simulink model "psb3levelVSC"  (Simulink 6.0)
settings: Solver=FixedStepDiscrete  SolverMode=SingleTasking  StartTime=0.0  StopTime=0.15  FixedStep=Ts_Power  RelTol=1e-3
PreLoadFcn:
  | assignin('base','Ts_Power',[5e-6]);assignin('base','Ts_Control',[100e-6])
undefined symbols (not defined in the file or in its folder): D1, Delta, gcbh, level, powericon, Ts_Control, Ts_Power
libraries: powerlib_extras x18, powerlib2 x17, simulink_extras x1
settings Model: Creator=sybille  LastModifiedBy=batserve  ExtModeTrigMode=oneshot  ExtModeArmWhenConnect=off  ExtModeAutoUpdateStatusClock=off  ProdHWDeviceType=Specified
settings DataIOCC: LimitDataPoints=off  SaveFormat=StructureWithTime  SaveOutput=off  SaveTime=off  SignalLoggingName=sigsOut
settings OptimizationCC: BlockReduction=off  BooleanDataType=off
settings DebuggingCC: SolverPrmCheckMsg=none
settings HardwareCC: ProdBitPerShort=32  ProdBitPerInt=16  ProdHWDeviceType=Specified  TargetUnknown=on

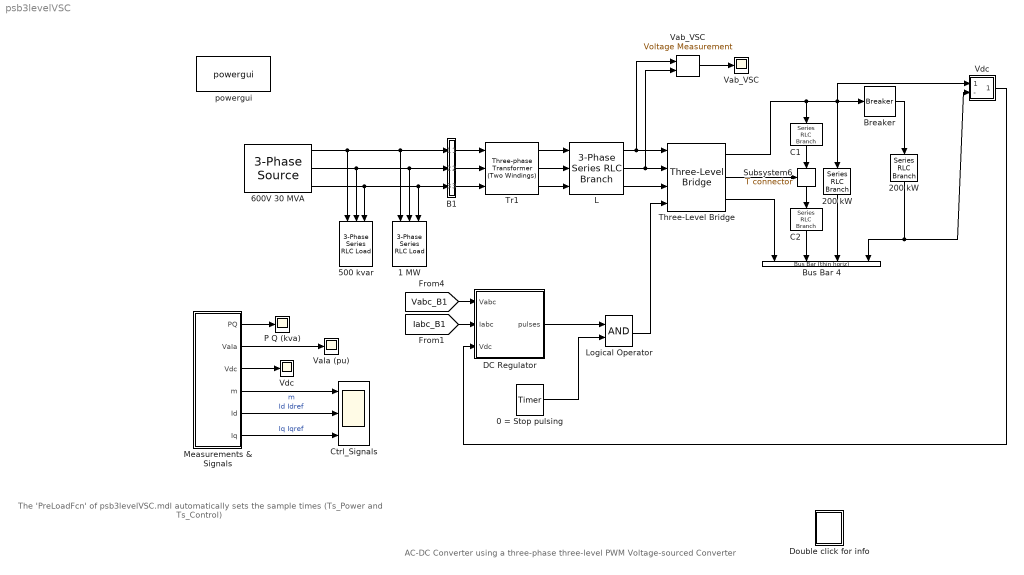
== system psb3levelVSC ==
  note: AC-DC Converter
      | using a three-phase three-level PWM Voltage-sourced Converter
  note: The 'PreLoadFcn' of psb3levelVSC.mdl automatically
      | sets the sample times (Ts_Power and Ts_Control)
  0 = Stop pulsing : powerlib_extras/Control  Blocks/Timer  t=[0 0.2]  e=[1 0]
  1 MW : powerlib2/Elements/3-Phase Series RLC Load  Orientation=down  Vpp=600  fn=60  P3=1e6  QL3=0  QC3=0
  200 kW : powerlib2/Elements/Series RLC Branch  Tag=PoWeRsYsTeMbLoCk  Orientation=down  a=500^2/200e3  b=0  c=inf  mesure=None  PSBOutputType=1
  "200 kW " : powerlib2/Elements/Series RLC Branch  Tag=PoWeRsYsTeMbLoCk  Orientation=down  a=500^2/200e3  b=0  c=inf  mesure=None  PSBOutputType=1
  500 kvar : powerlib2/Elements/3-Phase Series RLC Load  Orientation=down  Vpp=600  fn=60  P3=0.5e6/100  QL3=0  QC3=0.5e6
  600V 30 MVA : powerlib2/Electrical Sources/3-Phase Source  Tag=PoWeRsYsTeMbLoCk  V=600  Phi=0  F=60  InternalConnection=Yg  RLoff=on  R=0.724  L=19.2e-3  Psc=30e6  Vbase=600  XRratio=10  PSBOutputType=111
  B1 : Subsystem  Tag=PoWeRsYsTeMmEaSuReMeNt  AncestorBlock=powerlib2/Measurements/Three-Phase V-I Measurement  LoadFcn=powericon('psbloadfunction',gcbh,'3-Phase VI Measurement','');  InitFcn=powericon('checksum',bdroot)  mask(3-Phase VI Measurement){VChoice=phase-to-ground, ualv=on, labelV=Vabc_B1, Vpu=off, Vbase=500e3, IChoice=yes, ualc=on, labelC=Iabc_B1, Ppu=off, Pbase=100e6, OutputType=Magnitude, PhasorSimulation=off, PSBequivalent=0, PSBOutputType=11100}
      mask prompts: VChoice "Voltage measurement"; ualv "Use a label"; labelV "Signal label  (use a From block to collect signal)"; Vpu "Voltage  in pu"; Vbase "Base voltage (Vrms phase-phase) :"; IChoice "Current measurement"; ualc "Use a label"; labelC "Signal label  (use a From block to collect signal)"; Ppu "Currents in pu"; Pbase "Base power ( VA 3 phase)"; OutputType "Output signal :"; PhasorSimulation "Phasor simulation"; PSBequivalent "Equivalent circuit"
      mask help:
      | This block is used to measure three-phase voltages and currents in a circuit. When connected in series with a three-phase element, it return the three phase-to-ground voltages and line currents.
      |
      | The block can output the voltages and currents in per unit values or in volts and amperes. Check the appropriate boxes if you want to output the voltages and currents  in pu
      mask init:
      | powericon('psbcallbacks',gcb,'Three-phase measurements',4);
      | if  Vpu
      |     xKv=1/(Vbase/sqrt(3)*sqrt(2));
      | else
      |     xKv=1;
      | end
      | if  Ppu
      |     xKi=1/(Pbase/Vbase/sqrt(3)*sqrt(2));
      | else
      |     xKi=1;
      | end
      | switch OutputType
      | case 1
      |     OutputSelection  = [1:6];
      |     PhasorModeV = [1:3];
      |     NormalModeV = [7:9];
      |     PhasorModeI = [4:6];
      |     NormalModeI = [10:12];
      |     Kv = xKv;
      |     Ki = xKi;
      | case 2
      |     OutputSelection = [7,13,8,14,9,15,10,16,11,17,12,18];
      |     PhasorModeV = [1:6];
      |     NormalModeV = [13:15];
      |     PhasorModeI = [7:12];
      |     NormalModeI = [16:18];
      |     Kv = xKv;
      |     Ki = xKi;
      | case 3
      |     OutputSelection = [13,19,14,20,15,21,16,22,17,23,18,24];
      |     PhasorModeV = [1:6];
      |     NormalModeV = [13:15];
      |     PhasorModeI = [7:12];
      |     NormalModeI = [16:18];
      |     Kv = [xKv 1 xKv 1 xKv 1];
      |     Ki = [xKi 1 xKi 1 xKi 1];
      | case 4
      |     OutputSelection  = [19:24];
      |     PhasorModeV = [1:3];
      |     NormalModeV = [7:9];
      |     PhasorModeI = [4:6];
      |     NormalModeI = [10:12];
      |     Kv = xKv;
      |     Ki = xKi;
      | end
      | if PhasorSimulation
      |     SelectionModeV = PhasorModeV;
      |     SelectionModeI = PhasorModeI;
      | else
      |     SelectionModeV = NormalModeV;
      |     SelectionModeI = NormalModeI;
      |     Kv = xKv;
      |     Ki = xKi;
      | end
      settings: CopyFcn=powericon('psbloadfunction',gcbh,'3-Phase VI Measurement','VerifyPhasor');  CloseFcn=%3phaseVImeasurement
      mask Help: web(psbhelp)
      mask StyleString: popup(no|phase-to-ground|phase-to-phase),checkbox,edit,checkbox,edit,popup(no|yes),checkbox,edit,checkbox,edit,popup(Complex|Real-Imag|Magnitude-Angle|Magnitude),checkbox,edit,edit
      mask CallbackString: powericon('psbcallbacks',gcb,'Three-phase measurements',2);|powericon('psbcallbacks',gcb,'Three-phase measurements',2);||powericon('psbcallbacks',gcb,'Three-phase measurements',2);||powericon('psbcallbacks',gcb,'Three-phase measurements',2);|powericon('psbcallbacks',gcb,'Three-phase measurements',2);||powericon('psbcallbacks',gcb,'Three-phase measurements',4);|||||
  Breaker : powerlib2/Elements/Breaker  Tag=PoWeRsYsTeMbLoCk  a=0.001  c=0  rs=1e6  cs=inf  times=[0.15]  Ts=0  comext=off  mesure=None  PSBOutputType=1
  Bus Bar 4 : powerlib2/Connectors/Bus Bar (thin horiz)  Tag=PoWeRsYsTeMbLoCk  Orientation=down  input=4  output=0  PSBOutputType=111111111111111111111111111111111111111111111111111111111111111111111111111111111111
  C1 : powerlib2/Elements/Series RLC Branch  Tag=PoWeRsYsTeMbLoCk  Orientation=down  a=0  b=0  c=75000e-06  mesure=None  PSBOutputType=1
  C2 : powerlib2/Elements/Series RLC Branch  Tag=PoWeRsYsTeMbLoCk  Orientation=down  a=0  b=0  c=75000e-06  mesure=None  PSBOutputType=1
  Ctrl_Signals : Scope  NumInputPorts=3
      settings: YMin=0.6~-1~-1  YMax=1.2~1~1  SaveName=V_Load  DataFormat=Array  SampleInput=on  SampleTime=Ts_Control
  DC Regulator : Subsystem  mask(DC Voltage Regulator){Vdc_Ref=500}
      mask prompts: Vdc_Ref "DC voltage setpoint (V):"
  Double click for info : Subsystem
      mask Type: Information
      mask Display: disp('?')
  L : powerlib2/Elements/3-Phase Series RLC Branch   R=0.1e-3  L=20e-6  C=inf
  Logical Operator : Logic  AllPortsSameDT=off  OutDataTypeMode=Specify via dialog  LogicDataType=float('double')
  Measurements & Signals : Subsystem
  P Q (kva) : Scope
      settings: YMin=-25  YMax=425  SaveName=PQ  DataFormat=Array  SampleInput=on  SampleTime=Ts_Control
  Subsystem6 : powerlib2/Connectors/T connector  Tag=PoWeRsYsTeMbLoCk  Orientation=down  PSBOutputType=1
  Three-Level Bridge : powerlib2/Power Electronics/Three-Level Bridge  Tag=PoWeRsYsTeMbLoCk  arms=3  confi=ABC as input terminals  Rs=50  Cs=1e-6  device=IGBT / Diodes  Ron=0.2e-3  PAr_vf="[  2 1 ]"  mesure=All voltages and currents  PSBOutputType=111
  Tr1 : powerlib2/Elements/Three-phase Transformer (Two Windings)  Tag=PoWeRsYsTeMbLoCk  nominal=[ 500e3 , 60 ]  type1=Yg  params1=[ 600 , 0.04/30/2 , 0.04 ]  type2=Delta (D1)  params2=[ 240 , 0.04/30/2 , 0.0 ]  ynsat=off  rmag=500  lm=500  sat=[ 0,0 ; 0.0024,1.2 ; 1.0,1.52 ]  hyst=off  matfile='hysteresis'  sif=off  phi0=[ 0.8 , -0.8 , 0.7 ]  initialslopes=[+1 +1 +1]  mesure=None  PSBOutputType=1111
  VaIa (pu) : Scope
      settings: TimeRange=0.08  YMin=-2.5  YMax=1.5  SaveName=VaIa  SampleInput=on  SampleTime=Ts_Power*2
  Vab_VSC : Scope
      settings: TimeRange=0.05  YMin=-550  YMax=550  SaveName=Vab_VSC  SampleInput=on  SampleTime=Ts_Power
  "Vab_VSC " : powerlib2/Measurements/Voltage Measurement  Tag=PoWeRsYsTeMmEaSuReMeNt  PhasorSimulation=off  OutputType=Magnitude  PSBOutputType=0  PSBequivalent=0
  Vdc : Scope
      settings: YMin=200  YMax=600  SaveName=Vdc  DataFormat=Array  SampleInput=on  SampleTime=Ts_Control
  "Vdc " : Subsystem  Tag=PoWeRsYsTeMmEaSuReMeNt  AncestorBlock=powerlib2/Measurements/Voltage Measurement  LoadFcn=powericon('psblcfmeas',gcb)  InitFcn=powericon('checksum',bdroot)  mask(Voltage Measurement){PhasorSimulation=off, OutputType=Magnitude, PSBOutputType=0, PSBequivalent=0}
      mask prompts: PhasorSimulation "Phasor simulation"; OutputType "Output signal :"; PSBOutputType "Output type [1=PSB  0=simulink output]"; PSBequivalent "Equivalent circuit"
      mask help: Ideal voltage measurement.
      mask init:
      | switch OutputType
      | case 1
      |     OutputSelection = 1;
      |     NormalMode = 2;
      |     PhasorMode = 1;
      | case 2
      |     OutputSelection =[2,3];
      |     NormalMode = 3;
      |     PhasorMode = [1,2];
      | case 3
      |     OutputSelection =[4,5];
      |     NormalMode = 3;
      |     PhasorMode = [1,2];
      | case 4
      |     OutputSelection =[4];
      |     NormalMode = 2;
      |     PhasorMode = 1;
      | end
      | %
      | if PhasorSimulation
      |     SelectionMode = PhasorMode;
      | else
      |     SelectionMode = NormalMode;
      | end
      settings: CopyFcn=powericon('psblcfmeas',gcb,1)  ModelCloseFcn=powericon('loadsavedata',gcs,'close')
      mask Help: web(psbhelp);
      mask StyleString: checkbox,popup(Complex|Real-Imag|Magnitude-Angle|Magnitude),edit,edit
  powergui : powerlib2/powergui  Frange=logspace(0,3,50)  Ylog=off  Xlog=off  save=off  variable=ZData  structure=VaIa  ZoomFFT=on  StartTime=0.2  cycles=2  DisplayStyle=1  fundamental=60  FreqAxis=off  MaxFrequency=1000  frequencyindice=1  frequencyindicesteady=1  RmsSteady=2  display=off  Ts=Ts_Power  methode=off  frequency=60  echomessages=off
  wires:
  600V 30 MVA/1 -> B1/1(A), 1 MW/1, 500 kvar/1
  600V 30 MVA/2 -> B1/2(B), 1 MW/2, 500 kvar/2
  600V 30 MVA/3 -> B1/3(C), 1 MW/3, 500 kvar/3
  C1/1 -> Subsystem6/1
  Subsystem6/1 -> C2/1
  0 = Stop pulsing/1 -> Logical Operator/2
  DC Regulator/1(pulses) -> Logical Operator/1
  Tr1/1 -> L/1
  Tr1/2 -> L/2
  Tr1/3 -> L/3
  L/1 -> "Vab_VSC "/1, Three-Level Bridge/1
  L/2 -> Three-Level Bridge/2, "Vab_VSC "/2
  L/3 -> Three-Level Bridge/3
  Three-Level Bridge/2 -> Subsystem6/Enable
  Three-Level Bridge/1 -> "Vdc "/1(+), Breaker/1, 200 kW/1, C1/1
  C2/1 -> Bus Bar 4/2
  Three-Level Bridge/3 -> Bus Bar 4/1
  200 kW/1 -> Bus Bar 4/3
  Breaker/1 -> "200 kW "/1
  "200 kW "/1 -> "Vdc "/2(-), Bus Bar 4/4
  "Vab_VSC "/1 -> Vab_VSC/1
  Measurements & Signals/1(PQ) -> P Q (kva)/1
  Measurements & Signals/2(VaIa) -> VaIa (pu)/1
  Measurements & Signals/3(Vdc) -> Vdc/1
  Measurements & Signals/4(m) -> Ctrl_Signals/1  "m"
  Measurements & Signals/5(Id) -> Ctrl_Signals/2  "Id Idref"
  Measurements & Signals/6(Iq) -> Ctrl_Signals/3  "Iq Iqref"
  "Vdc "/1(v) -> DC Regulator/3(Vdc)
  B1/1("A ") -> Tr1/1
  B1/2("B ") -> Tr1/2
  B1/3("C ") -> Tr1/3
  [Vabc_B1] -> DC Regulator/1(Vabc)
  [Iabc_B1] -> DC Regulator/2(Iabc)
  Logical Operator/1 -> Three-Level Bridge/4

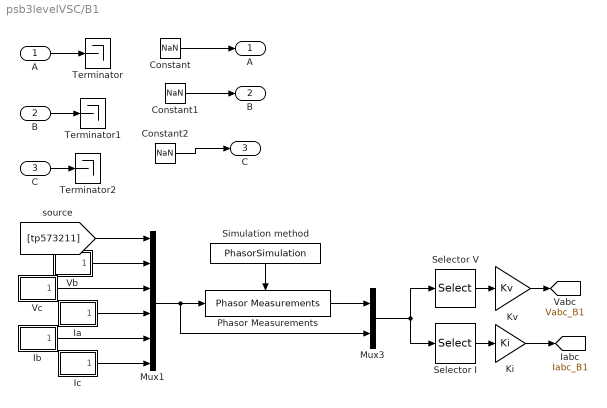
== system psb3levelVSC/B1 ==
  A : Inport  Port=1  LatchInput=off
  B : Inport  Port=2  LatchInput=off
  C : Inport  Port=3  LatchInput=off
  Constant : Constant  Value=NaN
  Constant1 : Constant  Value=NaN
  Constant2 : Constant  Value=NaN
  Ia : Subsystem  AncestorBlock=powerlib2/Measurements/Three-Phase V-I Measurement/Ia
  Ib : Subsystem  AncestorBlock=powerlib2/Measurements/Three-Phase V-I Measurement/Ib
  Ic : Subsystem  AncestorBlock=powerlib2/Measurements/Three-Phase V-I Measurement/Ic
  Ki : Gain  Gain=Ki  SaturateOnIntegerOverflow=on
  Kv : Gain  Gain=Kv  SaturateOnIntegerOverflow=on
  Mux1 : Mux  Inputs=6
  Mux3 : Mux  Inputs=2
  Phasor Measurements : powerlib2/Measurements/Three-Phase V-I Measurement/Phasor Measurements  TreatAsAtomicUnit=on  SimViewingDevice=off  DataTypeOverride=UseLocalSettings  MinMaxOverflowLogging=UseLocalSettings
      settings: Permissions=ReadWrite  RTWFcnNameOpts=Auto  RTWFileNameOpts=Auto
  Selector I : Selector  Elements=SelectionModeI  InputPortWidth=length(OutputSelection)+6
  Selector V : Selector  Elements=SelectionModeV  InputPortWidth=length(OutputSelection)+6
  Simulation method : Constant  Orientation=down  Value=PhasorSimulation
  Terminator : Terminator
  Terminator1 : Terminator
  Terminator2 : Terminator
  Vb : Subsystem  AncestorBlock=powerlib2/Measurements/Three-Phase V-I Measurement/Vb
  Vc : Subsystem  AncestorBlock=powerlib2/Measurements/Three-Phase V-I Measurement/Vc
  "A " : Outport
  "B " : Outport  Port=2
  "C " : Outport  Port=3
  tag scope: Iabc_B1=global, Vabc_B1=global
  wires:
  Ic/1(Out1) -> Mux1/6
  Ib/1(Out1) -> Mux1/5
  Ia/1(Out1) -> Mux1/4
  Vc/1(Out1) -> Mux1/3
  Vb/1(Out1) -> Mux1/2
  [tp573211] -> Mux1/1
  Mux1/1 -> Phasor Measurements/1, Mux3/2
  Simulation method/1 -> Phasor Measurements/Enable
  Phasor Measurements/1 -> Mux3/1
  Mux3/1 -> Selector V/1, Selector I/1
  Selector I/1 -> Ki/1
  Selector V/1 -> Kv/1
  Ki/1 -> [Iabc_B1]
  Kv/1 -> [Vabc_B1]
  Constant2/1 -> "C "/1
  Constant1/1 -> "B "/1
  Constant/1 -> "A "/1
  C/1 -> Terminator2/1
  B/1 -> Terminator1/1
  A/1 -> Terminator/1

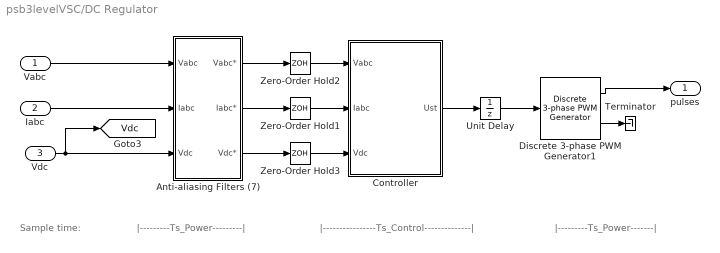
== system psb3levelVSC/DC Regulator ==
  note: |----------------Ts_Control--------------|
  note: |---------Ts_Power---------|
  note: Sample time:
  note: |---------Ts_Power-------|
  Vabc : Inport  Port=1  PortDimensions=3  LatchInput=off
  Iabc : Inport  Port=2  PortDimensions=3  LatchInput=off
  Vdc : Inport  Port=3  PortDimensions=1  LatchInput=off
  Anti-aliasing Filters (7) : Subsystem  mask(Anti-aliasing (2nd order lowpass)){Fc=750, Ts=Ts_Power}
      mask prompts: Fc "Cut-off frequency (Hz):"; Ts "Sample time:"
  Controller : Subsystem  mask(DC Regulator){Vdc_Ref=Vdc_Ref, Par_VdcReg=[0.015 1.6], Par_IReg=[0.3 20], Par_Nom=[600 500e3], Ts=Ts_Control}
      mask prompts: Vdc_Ref "DC Voltage setpoint (Volts)"; Par_VdcReg "Vdc Regulator Gains: [ Kp  Ki ]"; Par_IReg "Current Regulators Gain: [ Kp Ki Kd ]"; Par_Nom "Nominal Voltage and power: [ Vnom (volts rms L-L)  Pnom (VA) ]"; Ts "Time Step (s)"
      mask init:
      | Vnom=Par_Nom(1);
      | Pnom=Par_Nom(2);
      | Kp_I=Par_IReg(1);
      | Ki_I=Par_IReg(2);
      | Kp_Vdc=Par_VdcReg(1);
      | Ki_Vdc=Par_VdcReg(2);
  Discrete 3-phase PWM Generator1 : powerlib_extras/Discrete  Control Blocks/Discrete 3-phase PWM Generator  ModulatorType=3-level  ModulatorMode=Un-synchronized  nF=18  Fc=27*60  ModulatingSignals=off  m=0.2  Freq=60  Phase=0  Ts=Ts_Power
  Terminator : Terminator
  Unit Delay : UnitDelay  SampleTime=Ts_Control
  Zero-Order Hold1 : ZeroOrderHold  SampleTime=Ts_Control
  Zero-Order Hold2 : ZeroOrderHold  SampleTime=Ts_Control
  Zero-Order Hold3 : ZeroOrderHold  SampleTime=Ts_Control
  pulses : Outport
  tag scope: Vdc=global
  wires:
  Discrete 3-phase PWM Generator1/2 -> Terminator/1
  Discrete 3-phase PWM Generator1/1 -> pulses/1
  Unit Delay/1 -> Discrete 3-phase PWM Generator1/1
  Controller/1(Ust) -> Unit Delay/1
  Anti-aliasing Filters (7)/1(" Vabc*") -> Zero-Order Hold2/1
  Anti-aliasing Filters (7)/2(Iabc*) -> Zero-Order Hold1/1
  Anti-aliasing Filters (7)/3(" Vdc*") -> Zero-Order Hold3/1
  Zero-Order Hold3/1 -> Controller/3(Vdc)
  Zero-Order Hold1/1 -> Controller/2(Iabc)
  Zero-Order Hold2/1 -> Controller/1(Vabc)
  Vdc/1 -> [Vdc], Anti-aliasing Filters (7)/3("Vdc ")
  Iabc/1 -> Anti-aliasing Filters (7)/2("Iabc ")
  Vabc/1 -> Anti-aliasing Filters (7)/1(Vabc)

== system psb3levelVSC/Double click for info ==
  note: The DC regulator  uses two PI regulators to control the DC voltage while maintaining a unity input
      | power factor for the AC supply.
  note: 4) Controller:
  note: 2) AC Supply: three-phase, 600 V, 30 MVA, 60 Hz system
  note: 1) Converter rating: 500 Volts DC, 500 kW
  note: - DC Link: 2 capacitors of 75000 uF
  note: - Three-level, three-phase IGBT bridge (modeled using the "Three-Level Bridge" block)
      | controlled by a PWM modulator (carrier frequency of 1620 Hz)
  note: 3) Voltage-sourced Converter (VSC):
  note: Models Description:
  note: - In the simulation (lasting 150 ms), we can observe the following signals:
  note: Simulation Description:
  note: - Initial conditions set at the start of the simulation (by automatically loading the file: psb3levelVSC_xinit.mat prior to the simulation)
      | This file has been generated by running an initial simulation to steady-state for an integer number of cycles of 60 Hz.
      | The final states (both PSB and Simulink controllers states)  were saved in a vector, called xInitial. This vector, as
      | well as the sample times (Ts_Power and Ts_Control) were saved in "psb3levelVSC_xinit.mat" file
  note: Ts_Control= 100 us (used for the simulation of the DC regulator)
  note: - Two sample times: Ts_Power= 5 us (used by PSB for the simulation of the power system + converters)
  note: - Discrete (no continous states)
  note: AC-DC Converter
      | using a three-phase three-level PWM Voltage-sourced Converter
  note: Simulation Parameters:
  note: This AC-DC Converter demo illustrates the operation of the Three-Level Bridge block .
  note: P. Giroux ; G. Sybille Hydro-Quebec (IREQ)
  note: 1) the DC voltage (Vdc Scope)
      | 2) the primary voltage and current (phase A) of the AC supply (VaIa Scope),
      | 3) the device currents of leg A of the IGBT bridge (double-click inside the "Measurements & Signals" block to look inside the "Ia_Devices" Scope).
      | 4) the phase-to-phase AC voltage generated by the VSC (Vab_VSC Scope)
  note: - At 100 ms,  a "Stop Pulsing" signal is activated (pulses normally sent to the converter are blocked). We can see that the
      | DC voltage drops to 315 V. A drastic change in the primary current waveform can also be observed.
      | When the pulses are blocked, the Three-Level Bridge block operation becomes similar to a three-phase diode bridge.
  note: - At 50 ms, a 200-kW load is switched-in. We can see that the dynamic response of the DC regulator to this sudden load
      | variation (200 kW to 400 kW) is satisfactory. The DC voltage is back to 500 V within 1.5 cycle and the unity power factor
      | on the AC side is maintained.

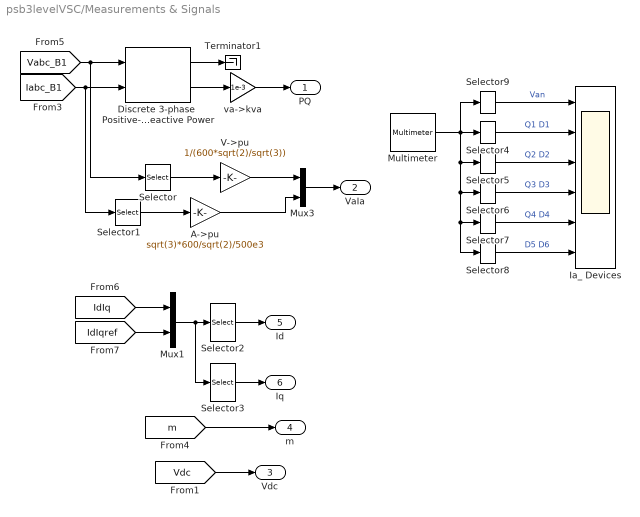
== system psb3levelVSC/Measurements & Signals ==
  A->pu : Gain  Gain=sqrt(3)*600/sqrt(2)/500e3  SaturateOnIntegerOverflow=on
  Discrete 3-phase  Positive-Sequence  Active & Reactive Power : powerlib_extras/Discrete Measurements/Discrete 3-phase  Positive-Sequence  Active & Reactive Power  Freq=60  Par_Vinit=[370 0]  Par_Iinit=[5 0]  Ts=Ts_Power
  Ia_ Devices : Scope  NumInputPorts=6
      settings: TimeRange=0.033  YMin=-400~-0~-0~0~0~0  YMax=300~7500~7500~4000~4000~7500  SaveName=I_Q3_disc1  DataFormat=Array  SampleInput=on  SampleTime=Ts_Power*2
  Multimeter : powerlib2/Measurements/Multimeter  Tag=PoWeRsYsTeMmEaSuReMeNt  PhasorSimulation=off  OutputType=Magnitude  sel=[1 6 7 8 9 10 11 12 13 14 15]  L=35  Gain=[1 1 1 1 1 1 1 1 1 1 1]  yselected={'Uan: Three-Level Bridge','IQ1a: Three-Level Bridge','IQ2a: Three-Level Bridge','IQ3a: Three-Level Bridge','IQ4a: Three-Level Bridge','ID1a: Three-Level Bridge','ID2a: Three-Level Bridge','ID3a: Three-Level Bridge','ID4a: Three-Level Bridge','ID5a: Three-Level Bridge','ID6a: Three-Level Bridge'};  PSBOutputType=1  PSBequivalent=0  AxesSetting=[0,0.1,-100,100]  Display=0  SavedBlockNames=-11
  Mux1 : Mux  Inputs=2
  Mux3 : Mux  Inputs=2
  Selector : Selector  InputPortWidth=3
  Selector1 : Selector  InputPortWidth=3
  Selector2 : Selector  Elements=[1 3]  InputPortWidth=4
  Selector3 : Selector  Elements=[1 3]+1  InputPortWidth=4
  Selector4 : Selector  Elements=[1 5]+1  InputPortWidth=11
  Selector5 : Selector  Elements=[1 5]+2  InputPortWidth=11
  Selector6 : Selector  Elements=[1 5]+3  InputPortWidth=11
  Selector7 : Selector  Elements=[1 5]+4  InputPortWidth=11
  Selector8 : Selector  Elements=[10 11]  InputPortWidth=11
  Selector9 : Selector  InputPortWidth=11
  Terminator1 : Terminator
  V->pu : Gain  Gain=1/(600*sqrt(2)/sqrt(3))  SaturateOnIntegerOverflow=on
  va->kva : Gain  Gain=1e-3  SaturateOnIntegerOverflow=on
  PQ : Outport
  VaIa : Outport  Port=2
  Vdc : Outport  Port=3
  m : Outport  Port=4
  Id : Outport  Port=5
  Iq : Outport  Port=6
  wires:
  va->kva/1 -> PQ/1
  Selector8/1 -> Ia_ Devices/6  "D5 D6"
  Selector7/1 -> Ia_ Devices/5  "Q4 D4"
  Selector6/1 -> Ia_ Devices/4  "Q3 D3"
  Selector5/1 -> Ia_ Devices/3  "Q2 D2"
  Selector4/1 -> Ia_ Devices/2  "Q1 D1"
  Multimeter/1 -> Selector9/1, Selector8/1, Selector7/1, Selector6/1, Selector5/1, Selector4/1
  Selector9/1 -> Ia_ Devices/1  "Van"
  A->pu/1 -> Mux3/2
  V->pu/1 -> Mux3/1
  Selector3/1 -> Iq/1
  Selector2/1 -> Id/1
  [m] -> m/1
  Mux1/1 -> Selector3/1, Selector2/1
  [Vdc] -> Vdc/1
  Mux3/1 -> VaIa/1
  Discrete 3-phase  Positive-Sequence  Active & Reactive Power/2 -> va->kva/1
  Discrete 3-phase  Positive-Sequence  Active & Reactive Power/1 -> Terminator1/1
  [Iabc_B1] -> Selector1/1, Discrete 3-phase  Positive-Sequence  Active & Reactive Power/2
  [Vabc_B1] -> Selector/1, Discrete 3-phase  Positive-Sequence  Active & Reactive Power/1
  Selector1/1 -> A->pu/1
  Selector/1 -> V->pu/1
  [IdIqref] -> Mux1/2
  [IdIq] -> Mux1/1

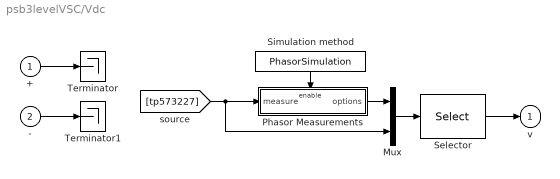
== system psb3levelVSC/Vdc  ==
  + : Inport  Port=1  LatchInput=off
  - : Inport  Port=2  LatchInput=off
  Mux : Mux  Inputs=2
  Phasor Measurements : Subsystem  TreatAsAtomicUnit=on
  Selector : Selector  Elements=SelectionMode  InputPortWidth=length(OutputSelection)+1
  Simulation method : Constant  Orientation=down  Value=PhasorSimulation
  Terminator : Terminator
  Terminator1 : Terminator
  v : Outport  InitialOutput=0
  wires:
  Simulation method/1 -> Phasor Measurements/Enable
  Mux/1 -> Selector/1
  Phasor Measurements/1(options) -> Mux/1
  Selector/1 -> v/1
  -/1 -> Terminator1/1
  +/1 -> Terminator/1
  [tp573227] -> Mux/2, Phasor Measurements/1(measure)

== system psb3levelVSC/B1/Ia ==
  Out1 : Outport
  wires:
  [tp573214] -> Out1/1

== system psb3levelVSC/B1/Ib ==
  Out1 : Outport
  wires:
  [tp573215] -> Out1/1

== system psb3levelVSC/B1/Ic ==
  Out1 : Outport
  wires:
  [tp573216] -> Out1/1

== system psb3levelVSC/B1/Vb ==
  Out1 : Outport
  wires:
  [tp573212] -> Out1/1

== system psb3levelVSC/B1/Vc ==
  Out1 : Outport
  wires:
  [tp573213] -> Out1/1

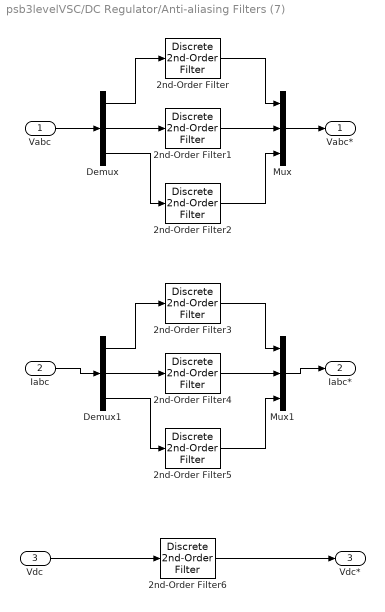
== system psb3levelVSC/DC Regulator/Anti-aliasing Filters (7) ==
  Vabc : Inport  Port=1  PortDimensions=3  LatchInput=off
  "Iabc " : Inport  Port=2  PortDimensions=3  LatchInput=off
  "Vdc " : Inport  Port=3  PortDimensions=1  LatchInput=off
  2nd-Order Filter : powerlib_extras/Discrete  Control Blocks/Discrete  2nd-Order Filter  FilterType=Lowpass  Fo=Fc  Zeta=0.707  Ts=Ts  Initialize=off  Vac_Init=[0.8 -25 60]  Vdc_Init=-0.4  PlotResponse=off  param1=[1 2000 0.2]
  2nd-Order Filter{1..2,4..6} (5 alike) : powerlib_extras/Discrete  Control Blocks/Discrete  2nd-Order Filter  FilterType=Lowpass  Fo=Fc  Zeta=0.707  Ts=Ts  Initialize=off  Vac_Init=[0.8 -25 60]  Vdc_Init=-0.4  PlotResponse=off  param1=[1 5000 0.1]
  2nd-Order Filter3 : powerlib_extras/Discrete  Control Blocks/Discrete  2nd-Order Filter  FilterType=Lowpass  Fo=Fc  Zeta=0.707  Ts=Ts  Initialize=off  Vac_Init=[0.8 -25 60]  Vdc_Init=-0.4  PlotResponse=off  param1=[1 2000 0.2]
  Demux : Demux  Outputs=3
  Demux1 : Demux  Outputs=3
  Mux : Mux  Inputs=3
  Mux1 : Mux  Inputs=3
  " Vabc*" : Outport
  Iabc* : Outport  Port=2
  " Vdc*" : Outport  Port=3
  wires:
  Mux1/1 -> Iabc*/1
  Demux1/2 -> 2nd-Order Filter4/1
  Demux1/3 -> 2nd-Order Filter5/1
  2nd-Order Filter5/1 -> Mux1/3
  2nd-Order Filter4/1 -> Mux1/2
  2nd-Order Filter3/1 -> Mux1/1
  Demux1/1 -> 2nd-Order Filter3/1
  "Iabc "/1 -> Demux1/1
  Demux/2 -> 2nd-Order Filter1/1
  Demux/3 -> 2nd-Order Filter2/1
  2nd-Order Filter2/1 -> Mux/3
  2nd-Order Filter1/1 -> Mux/2
  2nd-Order Filter6/1 -> " Vdc*"/1
  "Vdc "/1 -> 2nd-Order Filter6/1
  Mux/1 -> " Vabc*"/1
  2nd-Order Filter/1 -> Mux/1
  Vabc/1 -> Demux/1
  Demux/1 -> 2nd-Order Filter/1

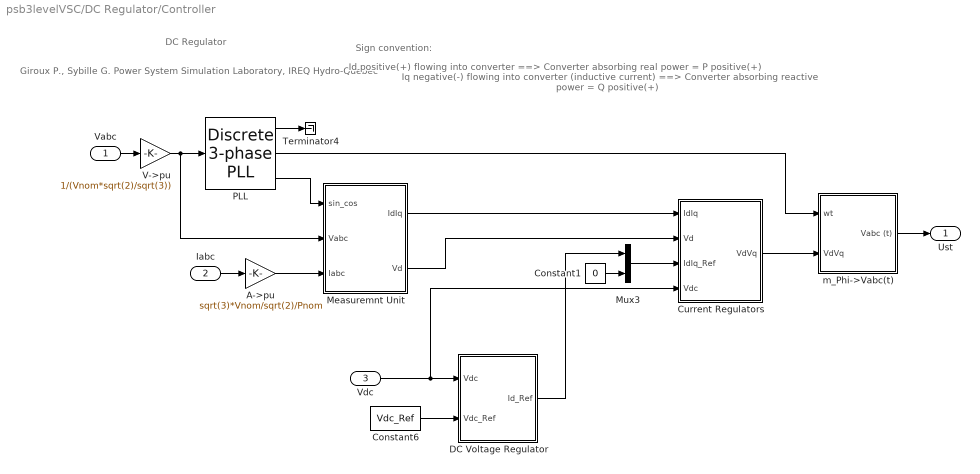
== system psb3levelVSC/DC Regulator/Controller ==
  note: DC Regulator
  note: Giroux P., Sybille G.
      | Power System Simulation Laboratory, IREQ
      | Hydro-Quebec
  note: Iq negative(-) flowing into converter (inductive current) ==> Converter absorbing reactive power = Q positive(+)
  note: Sign convention:
  note: Id positive(+) flowing into converter ==> Converter absorbing real power = P positive(+)
  Vabc : Inport  Port=1  PortDimensions=3  LatchInput=off
  Iabc : Inport  Port=2  PortDimensions=3  LatchInput=off
  Vdc : Inport  Port=3  PortDimensions=1  LatchInput=off
  A->pu : Gain  Gain=sqrt(3)*Vnom/sqrt(2)/Pnom  SaturateOnIntegerOverflow=on
  Constant1 : Constant  Value=0
  Constant6 : Constant  Value=Vdc_Ref
  Current Regulators : Subsystem  mask(Current Regulators){Kp=Kp_I, Ki=Ki_I, Kd=0, TcD=0.2e-3, Par_Limits=[12 -12], Init=0, Ts=Ts}
      mask prompts: Kp "Proportional gain (Kp):"; Ki "Integral gain (Ki):"; Kd "Derivative gain (Kd):"; TcD "Time constant for derivative (s):"; Par_Limits "Output limits: [ Upper   Lower ]"; Init "Output initial value:"; Ts "Sample time:"
      mask help:
      | Sign convention:
      | Id positive(+) flowing into converter ==> Converter absorbing real power = P positive(+)
      | Iq negative(-) flowing into converter (inductive current) ==> Converter absorbing reactive power = Q positive(+)
  DC Voltage Regulator : Subsystem  mask(DC Voltage regulator){Kp=Kp_Vdc, Ki=Ki_Vdc, Ts=Ts}
      mask prompts: Kp "Proportional gain (Kp):"; Ki "Integral gain(Ki)"; Ts "Sample time:"
  Measuremnt Unit : Subsystem
  Mux3 : Mux  Inputs=2
  PLL : powerlib_extras/Discrete  Control Blocks/Discrete 3-phase PLL  Fmin=45  Par_Init=[-45 60]  ParK=[60 1400]  Ts=Ts
  Terminator4 : Terminator
  V->pu : Gain  Gain=1/(Vnom*sqrt(2)/sqrt(3))  SaturateOnIntegerOverflow=on
  m_Phi->Vabc(t) : Subsystem
  Ust : Outport
  wires:
  m_Phi->Vabc(t)/1(Vabc (t)) -> Ust/1
  PLL/2 -> m_Phi->Vabc(t)/1(wt)
  Current Regulators/1(VdVq) -> m_Phi->Vabc(t)/2(VdVq)
  DC Voltage Regulator/1(Id_Ref) -> Mux3/1
  Constant1/1 -> Mux3/2
  Mux3/1 -> Current Regulators/3(IdIq_Ref)
  Measuremnt Unit/2(Vd) -> Current Regulators/2(Vd)
  Measuremnt Unit/1(IdIq) -> Current Regulators/1(IdIq)
  Iabc/1 -> A->pu/1
  PLL/3 -> Measuremnt Unit/1(sin_cos)
  PLL/1 -> Terminator4/1
  Vdc/1 -> Current Regulators/4(Vdc), DC Voltage Regulator/1(Vdc)
  Constant6/1 -> DC Voltage Regulator/2(Vdc_Ref)
  Vabc/1 -> V->pu/1
  V->pu/1 -> PLL/1, Measuremnt Unit/2(Vabc)
  A->pu/1 -> Measuremnt Unit/3(Iabc)

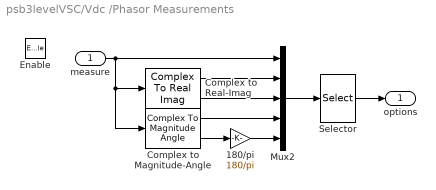
== system psb3levelVSC/Vdc /Phasor Measurements ==
  measure : Inport  Port=1  LatchInput=off
  Enable : EnablePort
  180/pi : Gain  Gain=180/pi  SaturateOnIntegerOverflow=on
  Complex to Magnitude-Angle : ComplexToMagnitudeAngle
  Complex to Real-Imag : ComplexToRealImag
  Mux2 : Mux  Inputs=5
  Selector : Selector  Elements=OutputSelection  InputPortWidth=5
  options : Outport  InitialOutput=0
  wires:
  Mux2/1 -> Selector/1
  measure/1 -> Complex to Magnitude-Angle/1, Complex to Real-Imag/1, Mux2/1
  Complex to Real-Imag/1 -> Mux2/2
  Complex to Real-Imag/2 -> Mux2/3
  Complex to Magnitude-Angle/1 -> Mux2/4
  Complex to Magnitude-Angle/2 -> 180/pi/1
  180/pi/1 -> Mux2/5
  Selector/1 -> options/1

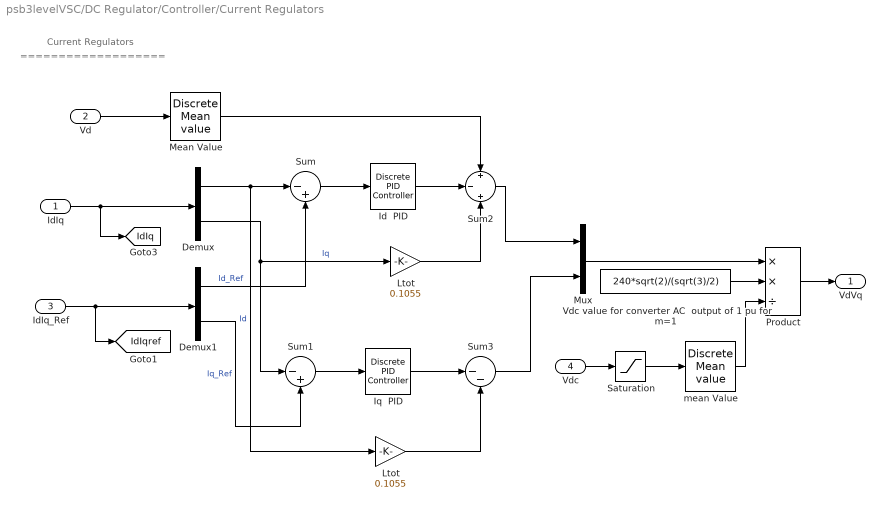
== system psb3levelVSC/DC Regulator/Controller/Current Regulators ==
  note: ===================
  note: Current Regulators
  IdIq : Inport  Port=1  PortDimensions=2  LatchInput=off
  Vd : Inport  Port=2  LatchInput=off
  IdIq_Ref : Inport  Port=3  PortDimensions=2  LatchInput=off
  Vdc : Inport  Port=4  LatchInput=off
  " Ltot" : Gain  Gain=0.1055  SaturateOnIntegerOverflow=on
  Demux : Demux  Outputs=2
  Demux1 : Demux  Outputs=2
  Id  PID : powerlib_extras/Discrete  Control Blocks/Discrete PID Controller  Kp=Kp  Ki=Ki  Kd=Kd  TcD=TcD  Par_Limits=Par_Limits  Init=Init  Ts=Ts
  Iq  PID : powerlib_extras/Discrete  Control Blocks/Discrete PID Controller  Kp=Kp  Ki=Ki  Kd=Kd  TcD=TcD  Par_Limits=Par_Limits  Init=Init  Ts=Ts
  "Ltot " : Gain  Gain=0.1055  SaturateOnIntegerOverflow=on
  Mean Value : powerlib_extras/Discrete Measurements/Discrete  Mean value  AncestorBlock=|  Freq=60  Vinit=1.007  Ts=Ts
      | powerlib_extras/Discrete
      | Measurements/Discrete 
      | Mean value
  Mux : Mux  Inputs=2
  Product : Product  Inputs=**/  SaturateOnIntegerOverflow=on  InputSameDT=on
  Saturation : Saturate  UpperLimit=10000  LowerLimit=10
  Sum : Sum  Inputs=|-+  SaturateOnIntegerOverflow=on  InputSameDT=on
  Sum1 : Sum  Inputs=|-+  SaturateOnIntegerOverflow=on  InputSameDT=on
  Sum2 : Sum  Inputs=+|-|+  SaturateOnIntegerOverflow=on  InputSameDT=on
  Sum3 : Sum  Inputs=|--  SaturateOnIntegerOverflow=on  InputSameDT=on
  Vdc value for converter AC  output of 1 pu for m=1 : Constant  Value=240*sqrt(2)/(sqrt(3)/2)
  "mean Value " : powerlib_extras/Discrete Measurements/Discrete  Mean value  AncestorBlock=|  Freq=60  Vinit=500  Ts=Ts
      | powerlib_extras/Discrete
      | Measurements/Discrete 
      | Mean value
  VdVq : Outport
  tag scope: IdIq=global, IdIqref=global
  wires:
  Sum3/1 -> Mux/2
  Vdc/1 -> Saturation/1
  "mean Value "/1 -> Product/3
  Vdc value for converter AC  output of 1 pu for m=1/1 -> Product/2
  Saturation/1 -> "mean Value "/1
  Mean Value/1 -> Sum2/1
  Product/1 -> VdVq/1
  IdIq_Ref/1 -> [IdIqref], Demux1/1
  Mux/1 -> Product/1
  Sum/1 -> Id  PID/1
  Demux1/2 -> Sum1/2  "Iq_Ref"
  Sum1/1 -> Iq  PID/1
  Demux/2 -> Sum1/1, "Ltot "/1  "Iq"
  Demux1/1 -> Sum/2  "Id_Ref"
  Demux/1 -> " Ltot"/1, Sum/1  "Id"
  IdIq/1 -> [IdIq], Demux/1
  Id  PID/1 -> Sum2/2
  Sum2/1 -> Mux/1
  Iq  PID/1 -> Sum3/1
  "Ltot "/1 -> Sum2/3
  " Ltot"/1 -> Sum3/2
  Vd/1 -> Mean Value/1

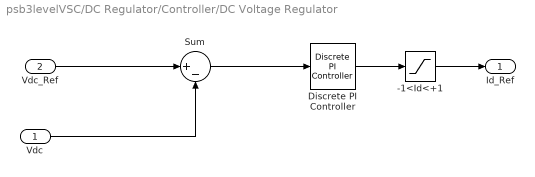
== system psb3levelVSC/DC Regulator/Controller/DC Voltage Regulator ==
  Vdc : Inport  Port=1  LatchInput=off
  Vdc_Ref : Inport  Port=2  LatchInput=off
  -1<Id<+1 : Saturate  UpperLimit=1.2  LowerLimit=-1.2
  Discrete PI Controller : powerlib_extras/Discrete  Control Blocks/Discrete PI Controller  Kp=Kp  Ki=Ki  Par_Limits=[1.2 -1.2]  Init=0  Ts=Ts
  Sum : Sum  Inputs=|+-  SaturateOnIntegerOverflow=on  InputSameDT=on
  Id_Ref : Outport  InitialOutput=0
  wires:
  Sum/1 -> Discrete PI Controller/1
  Vdc/1 -> Sum/2
  Discrete PI Controller/1 -> -1<Id<+1/1
  -1<Id<+1/1 -> Id_Ref/1
  Vdc_Ref/1 -> Sum/1

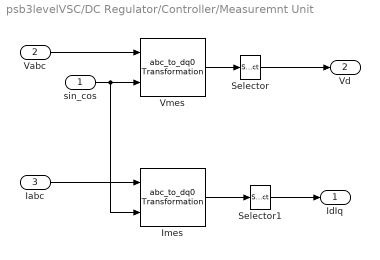
== system psb3levelVSC/DC Regulator/Controller/Measuremnt Unit ==
  sin_cos : Inport  Port=1  LatchInput=off
  Vabc : Inport  Port=2  LatchInput=off
  Iabc : Inport  Port=3  LatchInput=off
  Imes : powerlib_extras/Measurements/abc_to_dq0 Transformation
  Selector : Selector  InputPortWidth=3
  Selector1 : Selector  Elements=[1 2]  InputPortWidth=3
  Vmes : powerlib_extras/Measurements/abc_to_dq0 Transformation
  IdIq : Outport
  Vd : Outport  Port=2
  wires:
  Selector/1 -> Vd/1
  Imes/1 -> Selector1/1
  Iabc/1 -> Imes/1
  sin_cos/1 -> Imes/2, Vmes/2
  Vmes/1 -> Selector/1
  Vabc/1 -> Vmes/1
  Selector1/1 -> IdIq/1

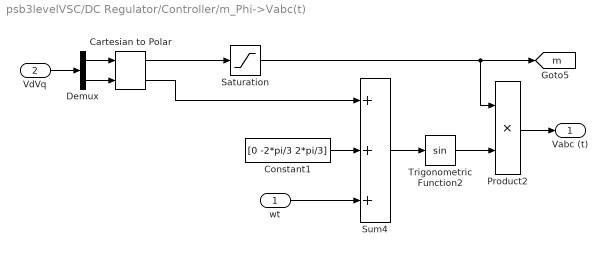
== system psb3levelVSC/DC Regulator/Controller/m_Phi->Vabc(t) ==
  wt : Inport  Port=1  LatchInput=off
  VdVq : Inport  Port=2  LatchInput=off
  Cartesian to Polar : simulink_extras/Transformations/Cartesian to Polar
  Constant1 : Constant  Value=[0 -2*pi/3 2*pi/3]
  Demux : Demux  Outputs=2
  Product2 : Product  SaturateOnIntegerOverflow=on  InputSameDT=on
  Saturation : Saturate  UpperLimit=1  LowerLimit=0
  Sum4 : Sum  Inputs=+++  SaturateOnIntegerOverflow=on  InputSameDT=on
  Trigonometric Function2 : Trigonometry
  Vabc (t) : Outport
  tag scope: m=global
  wires:
  Saturation/1 -> [m], Product2/1
  Cartesian to Polar/1 -> Saturation/1
  Trigonometric Function2/1 -> Product2/2
  Sum4/1 -> Trigonometric Function2/1
  Cartesian to Polar/2 -> Sum4/1
  Demux/2 -> Cartesian to Polar/2
  Demux/1 -> Cartesian to Polar/1
  VdVq/1 -> Demux/1
  wt/1 -> Sum4/3
  Product2/1 -> Vabc (t)/1
  Constant1/1 -> Sum4/2
